simulink model "assignment4"  (R2014a)
settings: Solver=VariableStepDiscrete  StartTime=0.0  StopTime=100000  RelTol=1e-3
libraries: hdlsllib x20, simulink x10
settings Model: Creator=hirn.j  LastModifiedBy=you.r
settings OptimizationCC: BlockReduction=off  ConditionallyExecuteInputs=off  InlineParams=on
settings DebuggingCC: AlgebraicLoopMsg=error
settings HardwareCC: ProdHWDeviceType=ASIC/FPGA->ASIC/FPGA  ProdEqTarget=off

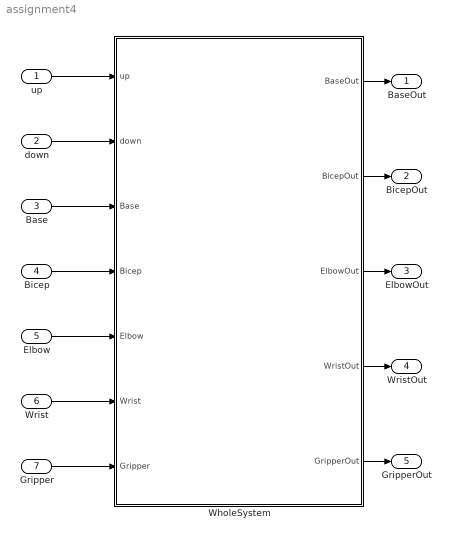
== system assignment4 ==
  up : Inport  OutDataTypeStr=boolean  SampleTime=1
  down : Inport  Port=2  OutDataTypeStr=boolean  SampleTime=1
  Base : Inport  Port=3  OutDataTypeStr=boolean  SampleTime=1
  Bicep : Inport  Port=4  OutDataTypeStr=boolean  SampleTime=1
  Elbow : Inport  Port=5  OutDataTypeStr=boolean  SampleTime=1
  Wrist : Inport  Port=6  OutDataTypeStr=boolean  SampleTime=1
  Gripper : Inport  Port=7  OutDataTypeStr=boolean  SampleTime=1
  WholeSystem : Subsystem  TreatAsAtomicUnit=on  SystemSampleTime=1
  BaseOut : Outport  SampleTime=1
  BicepOut : Outport  Port=2  SampleTime=1
  ElbowOut : Outport  Port=3  SampleTime=1
  WristOut : Outport  Port=4  SampleTime=1
  GripperOut : Outport  Port=5  SampleTime=1
  wires:
  up/1 -> WholeSystem/1(up)
  down/1 -> WholeSystem/2(down)
  Base/1 -> WholeSystem/3(Base)
  Bicep/1 -> WholeSystem/4(Bicep)
  Elbow/1 -> WholeSystem/5(Elbow)
  Wrist/1 -> WholeSystem/6(Wrist)
  Gripper/1 -> WholeSystem/7(Gripper)
  WholeSystem/1(BaseOut) -> BaseOut/1
  WholeSystem/2(BicepOut) -> BicepOut/1
  WholeSystem/3(ElbowOut) -> ElbowOut/1
  WholeSystem/4(WristOut) -> WristOut/1
  WholeSystem/5(GripperOut) -> GripperOut/1

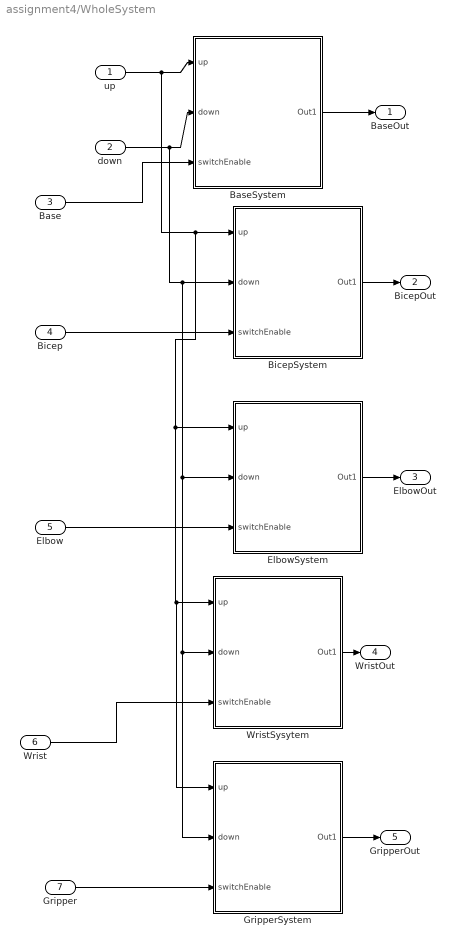
== system assignment4/WholeSystem ==
  up : Inport  OutDataTypeStr=boolean  SampleTime=1
  down : Inport  Port=2  OutDataTypeStr=boolean  SampleTime=1
  Base : Inport  Port=3  OutDataTypeStr=boolean  SampleTime=1
  Bicep : Inport  Port=4  OutDataTypeStr=boolean  SampleTime=1
  Elbow : Inport  Port=5  OutDataTypeStr=boolean  SampleTime=1
  Wrist : Inport  Port=6  OutDataTypeStr=boolean  SampleTime=1
  Gripper : Inport  Port=7  OutDataTypeStr=boolean  SampleTime=1
  BaseSystem : Subsystem  TreatAsAtomicUnit=on  SystemSampleTime=1
  BicepSystem : Subsystem  TreatAsAtomicUnit=on  SystemSampleTime=1
  ElbowSystem : Subsystem  TreatAsAtomicUnit=on  SystemSampleTime=1
  GripperSystem : Subsystem  TreatAsAtomicUnit=on  SystemSampleTime=1
  WristSysytem : Subsystem  TreatAsAtomicUnit=on  SystemSampleTime=1
  BaseOut : Outport  SampleTime=1
  BicepOut : Outport  Port=2  SampleTime=1
  ElbowOut : Outport  Port=3  SampleTime=1
  WristOut : Outport  Port=4  SampleTime=1
  GripperOut : Outport  Port=5  SampleTime=1
  wires:
  GripperSystem/1(Out1) -> GripperOut/1
  Bicep/1 -> BicepSystem/3(switchEnable)
  Base/1 -> BaseSystem/3(switchEnable)
  Wrist/1 -> WristSysytem/3(switchEnable)
  Elbow/1 -> ElbowSystem/3(switchEnable)
  Gripper/1 -> GripperSystem/3(switchEnable)
  up/1 -> GripperSystem/1(up), WristSysytem/1(up), ElbowSystem/1(up), BicepSystem/1(up), BaseSystem/1(up)
  down/1 -> GripperSystem/2(down), WristSysytem/2(down), ElbowSystem/2(down), BicepSystem/2(down), BaseSystem/2(down)
  BaseSystem/1(Out1) -> BaseOut/1
  BicepSystem/1(Out1) -> BicepOut/1
  WristSysytem/1(Out1) -> WristOut/1
  ElbowSystem/1(Out1) -> ElbowOut/1

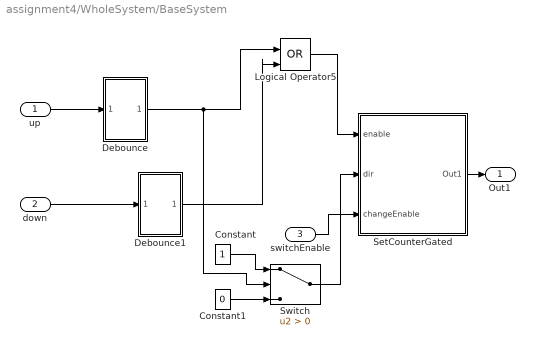
== system assignment4/WholeSystem/BaseSystem ==
  up : Inport  OutDataTypeStr=boolean  SampleTime=1
  down : Inport  Port=2  OutDataTypeStr=boolean  SampleTime=1
  switchEnable : Inport  Port=3  OutDataTypeStr=boolean  SampleTime=1
  Constant : Constant  OutDataTypeStr=boolean
  Constant1 : Constant  Value=0  OutDataTypeStr=boolean
  Debounce : Subsystem
  Debounce1 : Subsystem
  Logical Operator5 : Logic  Operator=OR  IconShape=distinctive  AllPortsSameDT=off  OutDataTypeStr=boolean  SampleTime=1
  SetCounterGated : Subsystem
  Switch : Switch  Criteria=u2 > Threshold
  Out1 : Outport  SampleTime=1
  wires:
  Debounce/1(Out1) -> Switch/2, Logical Operator5/1
  Logical Operator5/1 -> SetCounterGated/1(enable)
  up/1 -> Debounce/1(In1)
  down/1 -> Debounce1/1(In1)
  Constant/1 -> Switch/1
  Switch/1 -> SetCounterGated/2(dir)
  Constant1/1 -> Switch/3
  Debounce1/1(Out1) -> Logical Operator5/2
  SetCounterGated/1(Out1) -> Out1/1
  switchEnable/1 -> SetCounterGated/3(changeEnable)

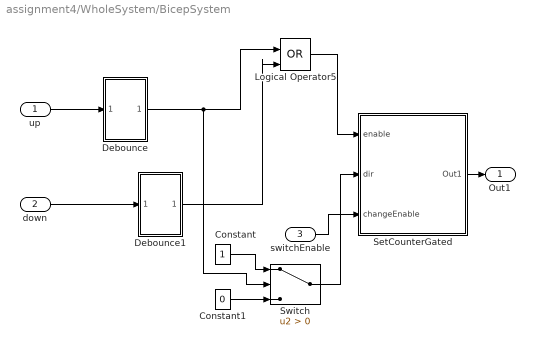
== system assignment4/WholeSystem/BicepSystem ==
  up : Inport  OutDataTypeStr=boolean  SampleTime=1
  down : Inport  Port=2  OutDataTypeStr=boolean  SampleTime=1
  switchEnable : Inport  Port=3  OutDataTypeStr=boolean  SampleTime=1
  Constant : Constant  OutDataTypeStr=boolean
  Constant1 : Constant  Value=0  OutDataTypeStr=boolean
  Debounce : Subsystem
  Debounce1 : Subsystem
  Logical Operator5 : Logic  Operator=OR  IconShape=distinctive  AllPortsSameDT=off  OutDataTypeStr=boolean  SampleTime=1
  SetCounterGated : Subsystem
  Switch : Switch  Criteria=u2 > Threshold
  Out1 : Outport  SampleTime=1
  wires:
  Debounce/1(Out1) -> Switch/2, Logical Operator5/1
  Logical Operator5/1 -> SetCounterGated/1(enable)
  up/1 -> Debounce/1(In1)
  down/1 -> Debounce1/1(In1)
  Constant/1 -> Switch/1
  Switch/1 -> SetCounterGated/2(dir)
  Constant1/1 -> Switch/3
  Debounce1/1(Out1) -> Logical Operator5/2
  SetCounterGated/1(Out1) -> Out1/1
  switchEnable/1 -> SetCounterGated/3(changeEnable)

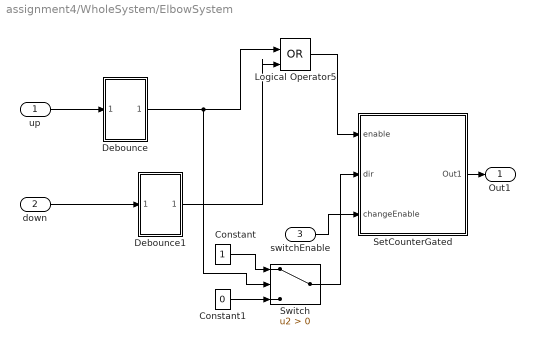
== system assignment4/WholeSystem/ElbowSystem ==
  up : Inport  OutDataTypeStr=boolean  SampleTime=1
  down : Inport  Port=2  OutDataTypeStr=boolean  SampleTime=1
  switchEnable : Inport  Port=3  OutDataTypeStr=boolean  SampleTime=1
  Constant : Constant  OutDataTypeStr=boolean
  Constant1 : Constant  Value=0  OutDataTypeStr=boolean
  Debounce : Subsystem
  Debounce1 : Subsystem
  Logical Operator5 : Logic  Operator=OR  IconShape=distinctive  AllPortsSameDT=off  OutDataTypeStr=boolean  SampleTime=1
  SetCounterGated : Subsystem
  Switch : Switch  Criteria=u2 > Threshold
  Out1 : Outport  SampleTime=1
  wires:
  Debounce/1(Out1) -> Switch/2, Logical Operator5/1
  Logical Operator5/1 -> SetCounterGated/1(enable)
  up/1 -> Debounce/1(In1)
  down/1 -> Debounce1/1(In1)
  Constant/1 -> Switch/1
  Switch/1 -> SetCounterGated/2(dir)
  Constant1/1 -> Switch/3
  Debounce1/1(Out1) -> Logical Operator5/2
  SetCounterGated/1(Out1) -> Out1/1
  switchEnable/1 -> SetCounterGated/3(changeEnable)

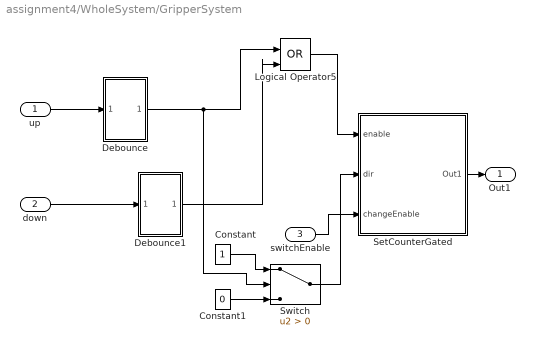
== system assignment4/WholeSystem/GripperSystem ==
  up : Inport  OutDataTypeStr=boolean  SampleTime=1
  down : Inport  Port=2  OutDataTypeStr=boolean  SampleTime=1
  switchEnable : Inport  Port=3  OutDataTypeStr=boolean  SampleTime=1
  Constant : Constant  OutDataTypeStr=boolean
  Constant1 : Constant  Value=0  OutDataTypeStr=boolean
  Debounce : Subsystem
  Debounce1 : Subsystem
  Logical Operator5 : Logic  Operator=OR  IconShape=distinctive  AllPortsSameDT=off  OutDataTypeStr=boolean  SampleTime=1
  SetCounterGated : Subsystem
  Switch : Switch  Criteria=u2 > Threshold
  Out1 : Outport  SampleTime=1
  wires:
  Debounce/1(Out1) -> Switch/2, Logical Operator5/1
  Logical Operator5/1 -> SetCounterGated/1(enable)
  up/1 -> Debounce/1(In1)
  down/1 -> Debounce1/1(In1)
  Constant/1 -> Switch/1
  Switch/1 -> SetCounterGated/2(dir)
  Constant1/1 -> Switch/3
  Debounce1/1(Out1) -> Logical Operator5/2
  SetCounterGated/1(Out1) -> Out1/1
  switchEnable/1 -> SetCounterGated/3(changeEnable)

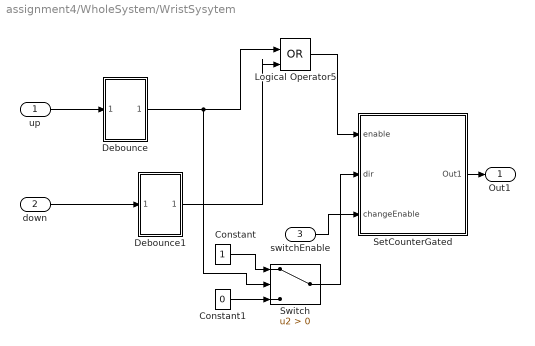
== system assignment4/WholeSystem/WristSysytem ==
  up : Inport  OutDataTypeStr=boolean  SampleTime=1
  down : Inport  Port=2  OutDataTypeStr=boolean  SampleTime=1
  switchEnable : Inport  Port=3  OutDataTypeStr=boolean  SampleTime=1
  Constant : Constant  OutDataTypeStr=boolean
  Constant1 : Constant  Value=0  OutDataTypeStr=boolean
  Debounce : Subsystem
  Debounce1 : Subsystem
  Logical Operator5 : Logic  Operator=OR  IconShape=distinctive  AllPortsSameDT=off  OutDataTypeStr=boolean  SampleTime=1
  SetCounterGated : Subsystem
  Switch : Switch  Criteria=u2 > Threshold
  Out1 : Outport  SampleTime=1
  wires:
  Debounce/1(Out1) -> Switch/2, Logical Operator5/1
  Logical Operator5/1 -> SetCounterGated/1(enable)
  up/1 -> Debounce/1(In1)
  down/1 -> Debounce1/1(In1)
  Constant/1 -> Switch/1
  Switch/1 -> SetCounterGated/2(dir)
  Constant1/1 -> Switch/3
  Debounce1/1(Out1) -> Logical Operator5/2
  SetCounterGated/1(Out1) -> Out1/1
  switchEnable/1 -> SetCounterGated/3(changeEnable)

== system assignment4/WholeSystem/BaseSystem/Debounce ==
  In1 : Inport
  Compare To Constant2 : simulink/Logic and Bit Operations/Compare To Constant  relop===  const=12500000  OutDataTypeStr=boolean
  Data Type Conversion1 : DataTypeConversion  OutDataTypeStr=boolean
  HDL Counter4 : hdlsllib/HDL Operations/HDL Counter  CountType=Free running  CountInit=0  CountStep=1  CountMax=100  CountFromType=Initial value  CountFrom=0  CountResetPort=on  CountLoadPort=off  CountEnbPort=on  CountDirPort=off  CountDataType=Unsigned  CountWordLen=32  CountFracLen=0  CountSampTime=1
  Logical Operator1 : Logic  Operator=NOT  IconShape=distinctive  AllPortsSameDT=off  OutDataTypeStr=boolean  SampleTime=1
  Out1 : Outport
  wires:
  Logical Operator1/1 -> HDL Counter4/1
  Compare To Constant2/1 -> Data Type Conversion1/1
  In1/1 -> HDL Counter4/2, Logical Operator1/1
  Data Type Conversion1/1 -> Out1/1
  HDL Counter4/1 -> Compare To Constant2/1

== system assignment4/WholeSystem/BaseSystem/Debounce1 ==
  In1 : Inport
  Compare To Constant2 : simulink/Logic and Bit Operations/Compare To Constant  relop===  const=12500000  OutDataTypeStr=boolean
  Data Type Conversion1 : DataTypeConversion  OutDataTypeStr=boolean
  HDL Counter4 : hdlsllib/HDL Operations/HDL Counter  CountType=Free running  CountInit=0  CountStep=1  CountMax=100  CountFromType=Initial value  CountFrom=0  CountResetPort=on  CountLoadPort=off  CountEnbPort=on  CountDirPort=off  CountDataType=Unsigned  CountWordLen=32  CountFracLen=0  CountSampTime=1
  Logical Operator1 : Logic  Operator=NOT  IconShape=distinctive  AllPortsSameDT=off  OutDataTypeStr=boolean  SampleTime=1
  Out1 : Outport
  wires:
  Logical Operator1/1 -> HDL Counter4/1
  Compare To Constant2/1 -> Data Type Conversion1/1
  In1/1 -> HDL Counter4/2, Logical Operator1/1
  Data Type Conversion1/1 -> Out1/1
  HDL Counter4/1 -> Compare To Constant2/1

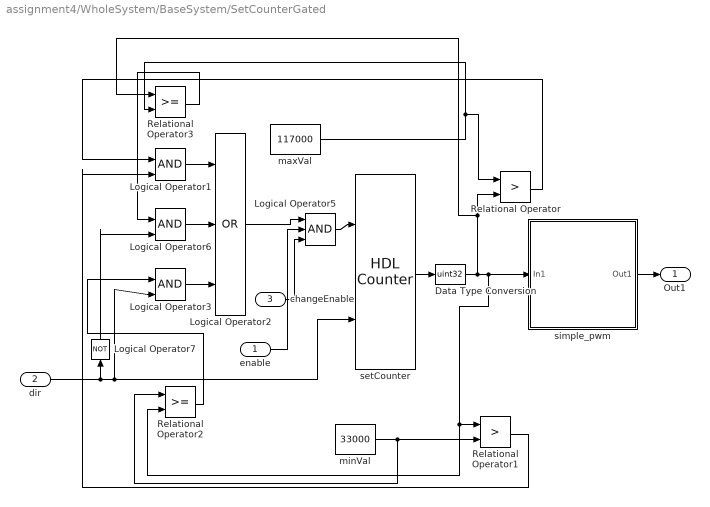
== system assignment4/WholeSystem/BaseSystem/SetCounterGated ==
  enable : Inport  OutDataTypeStr=boolean
  dir : Inport  Port=2  OutDataTypeStr=boolean
  changeEnable : Inport  Port=3  OutDataTypeStr=boolean
  Data Type Conversion : DataTypeConversion  OutDataTypeStr=uint32
  Logical Operator1 : Logic  IconShape=distinctive  AllPortsSameDT=off  OutDataTypeStr=boolean  SampleTime=1
  Logical Operator2 : Logic  Operator=OR  Inputs=3  IconShape=distinctive  AllPortsSameDT=off  OutDataTypeStr=boolean  SampleTime=1
  Logical Operator3 : Logic  IconShape=distinctive  AllPortsSameDT=off  OutDataTypeStr=boolean  SampleTime=1
  Logical Operator5 : Logic  Inputs=3  IconShape=distinctive  AllPortsSameDT=off  OutDataTypeStr=boolean  SampleTime=1
  Logical Operator6 : Logic  IconShape=distinctive  AllPortsSameDT=off  OutDataTypeStr=boolean  SampleTime=1
  Logical Operator7 : Logic  Operator=NOT  IconShape=distinctive  AllPortsSameDT=off  OutDataTypeStr=boolean  SampleTime=1
  Relational Operator : RelationalOperator  Operator=>  OutDataTypeStr=boolean
  Relational Operator1 : RelationalOperator  Operator=>  OutDataTypeStr=boolean
  Relational Operator2 : RelationalOperator  OutDataTypeStr=boolean
  Relational Operator3 : RelationalOperator  OutDataTypeStr=boolean
  maxVal : Constant  Value=117000  OutDataTypeStr=uint32
  minVal : Constant  Value=33000  OutDataTypeStr=uint32
  setCounter : hdlsllib/HDL Operations/HDL Counter  CountType=Count limited  CountInit=75000  CountStep=6000  CountMax=120000  CountFromType=Specify  CountFrom=30000  CountResetPort=off  CountLoadPort=off  CountEnbPort=on  CountDirPort=on  CountDataType=Unsigned  CountWordLen=20  CountFracLen=0  CountSampTime=1
  simple_pwm : Subsystem
  Out1 : Outport
  wires:
  Logical Operator7/1 -> Logical Operator6/2
  enable/1 -> Logical Operator5/2
  dir/1 -> Logical Operator7/1, Logical Operator3/2, setCounter/2
  setCounter/1 -> Data Type Conversion/1
  Logical Operator1/1 -> Logical Operator2/1
  Relational Operator/1 -> Logical Operator1/1
  maxVal/1 -> Relational Operator3/2, Relational Operator/1
  Logical Operator5/1 -> setCounter/1
  Relational Operator1/1 -> Logical Operator1/2
  Logical Operator2/1 -> Logical Operator5/1
  Logical Operator6/1 -> Logical Operator2/2
  Logical Operator3/1 -> Logical Operator2/3
  simple_pwm/1(Out1) -> Out1/1
  Data Type Conversion/1 -> Relational Operator2/2, Relational Operator1/1, simple_pwm/1(In1), Relational Operator3/1, Relational Operator/2
  minVal/1 -> Relational Operator2/1, Relational Operator1/2
  Relational Operator2/1 -> Logical Operator3/1
  Relational Operator3/1 -> Logical Operator6/1
  changeEnable/1 -> Logical Operator5/3

== system assignment4/WholeSystem/BicepSystem/Debounce ==
  In1 : Inport
  Compare To Constant2 : simulink/Logic and Bit Operations/Compare To Constant  relop===  const=12500000  OutDataTypeStr=boolean
  Data Type Conversion1 : DataTypeConversion  OutDataTypeStr=boolean
  HDL Counter4 : hdlsllib/HDL Operations/HDL Counter  CountType=Free running  CountInit=0  CountStep=1  CountMax=100  CountFromType=Initial value  CountFrom=0  CountResetPort=on  CountLoadPort=off  CountEnbPort=on  CountDirPort=off  CountDataType=Unsigned  CountWordLen=32  CountFracLen=0  CountSampTime=1
  Logical Operator1 : Logic  Operator=NOT  IconShape=distinctive  AllPortsSameDT=off  OutDataTypeStr=boolean  SampleTime=1
  Out1 : Outport
  wires:
  Logical Operator1/1 -> HDL Counter4/1
  Compare To Constant2/1 -> Data Type Conversion1/1
  In1/1 -> HDL Counter4/2, Logical Operator1/1
  Data Type Conversion1/1 -> Out1/1
  HDL Counter4/1 -> Compare To Constant2/1

== system assignment4/WholeSystem/BicepSystem/Debounce1 ==
  In1 : Inport
  Compare To Constant2 : simulink/Logic and Bit Operations/Compare To Constant  relop===  const=12500000  OutDataTypeStr=boolean
  Data Type Conversion1 : DataTypeConversion  OutDataTypeStr=boolean
  HDL Counter4 : hdlsllib/HDL Operations/HDL Counter  CountType=Free running  CountInit=0  CountStep=1  CountMax=100  CountFromType=Initial value  CountFrom=0  CountResetPort=on  CountLoadPort=off  CountEnbPort=on  CountDirPort=off  CountDataType=Unsigned  CountWordLen=32  CountFracLen=0  CountSampTime=1
  Logical Operator1 : Logic  Operator=NOT  IconShape=distinctive  AllPortsSameDT=off  OutDataTypeStr=boolean  SampleTime=1
  Out1 : Outport
  wires:
  Logical Operator1/1 -> HDL Counter4/1
  Compare To Constant2/1 -> Data Type Conversion1/1
  In1/1 -> HDL Counter4/2, Logical Operator1/1
  Data Type Conversion1/1 -> Out1/1
  HDL Counter4/1 -> Compare To Constant2/1

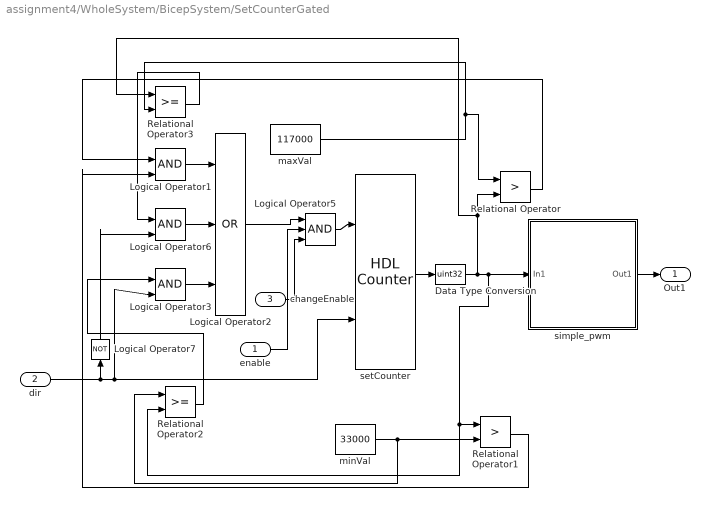
== system assignment4/WholeSystem/BicepSystem/SetCounterGated ==
  enable : Inport  OutDataTypeStr=boolean
  dir : Inport  Port=2  OutDataTypeStr=boolean
  changeEnable : Inport  Port=3  OutDataTypeStr=boolean
  Data Type Conversion : DataTypeConversion  OutDataTypeStr=uint32
  Logical Operator1 : Logic  IconShape=distinctive  AllPortsSameDT=off  OutDataTypeStr=boolean  SampleTime=1
  Logical Operator2 : Logic  Operator=OR  Inputs=3  IconShape=distinctive  AllPortsSameDT=off  OutDataTypeStr=boolean  SampleTime=1
  Logical Operator3 : Logic  IconShape=distinctive  AllPortsSameDT=off  OutDataTypeStr=boolean  SampleTime=1
  Logical Operator5 : Logic  Inputs=3  IconShape=distinctive  AllPortsSameDT=off  OutDataTypeStr=boolean  SampleTime=1
  Logical Operator6 : Logic  IconShape=distinctive  AllPortsSameDT=off  OutDataTypeStr=boolean  SampleTime=1
  Logical Operator7 : Logic  Operator=NOT  IconShape=distinctive  AllPortsSameDT=off  OutDataTypeStr=boolean  SampleTime=1
  Relational Operator : RelationalOperator  Operator=>  OutDataTypeStr=boolean
  Relational Operator1 : RelationalOperator  Operator=>  OutDataTypeStr=boolean
  Relational Operator2 : RelationalOperator  OutDataTypeStr=boolean
  Relational Operator3 : RelationalOperator  OutDataTypeStr=boolean
  maxVal : Constant  Value=117000  OutDataTypeStr=uint32
  minVal : Constant  Value=33000  OutDataTypeStr=uint32
  setCounter : hdlsllib/HDL Operations/HDL Counter  CountType=Count limited  CountInit=75000  CountStep=6000  CountMax=120000  CountFromType=Specify  CountFrom=30000  CountResetPort=off  CountLoadPort=off  CountEnbPort=on  CountDirPort=on  CountDataType=Unsigned  CountWordLen=20  CountFracLen=0  CountSampTime=1
  simple_pwm : Subsystem
  Out1 : Outport
  wires:
  Logical Operator7/1 -> Logical Operator6/2
  enable/1 -> Logical Operator5/2
  dir/1 -> Logical Operator7/1, Logical Operator3/2, setCounter/2
  setCounter/1 -> Data Type Conversion/1
  Logical Operator1/1 -> Logical Operator2/1
  Relational Operator/1 -> Logical Operator1/1
  maxVal/1 -> Relational Operator3/2, Relational Operator/1
  Logical Operator5/1 -> setCounter/1
  Relational Operator1/1 -> Logical Operator1/2
  Logical Operator2/1 -> Logical Operator5/1
  Logical Operator6/1 -> Logical Operator2/2
  Logical Operator3/1 -> Logical Operator2/3
  simple_pwm/1(Out1) -> Out1/1
  Data Type Conversion/1 -> Relational Operator2/2, Relational Operator1/1, simple_pwm/1(In1), Relational Operator3/1, Relational Operator/2
  minVal/1 -> Relational Operator2/1, Relational Operator1/2
  Relational Operator2/1 -> Logical Operator3/1
  Relational Operator3/1 -> Logical Operator6/1
  changeEnable/1 -> Logical Operator5/3

== system assignment4/WholeSystem/ElbowSystem/Debounce ==
  In1 : Inport
  Compare To Constant2 : simulink/Logic and Bit Operations/Compare To Constant  relop===  const=12500000  OutDataTypeStr=boolean
  Data Type Conversion1 : DataTypeConversion  OutDataTypeStr=boolean
  HDL Counter4 : hdlsllib/HDL Operations/HDL Counter  CountType=Free running  CountInit=0  CountStep=1  CountMax=100  CountFromType=Initial value  CountFrom=0  CountResetPort=on  CountLoadPort=off  CountEnbPort=on  CountDirPort=off  CountDataType=Unsigned  CountWordLen=32  CountFracLen=0  CountSampTime=1
  Logical Operator1 : Logic  Operator=NOT  IconShape=distinctive  AllPortsSameDT=off  OutDataTypeStr=boolean  SampleTime=1
  Out1 : Outport
  wires:
  Logical Operator1/1 -> HDL Counter4/1
  Compare To Constant2/1 -> Data Type Conversion1/1
  In1/1 -> HDL Counter4/2, Logical Operator1/1
  Data Type Conversion1/1 -> Out1/1
  HDL Counter4/1 -> Compare To Constant2/1

== system assignment4/WholeSystem/ElbowSystem/Debounce1 ==
  In1 : Inport
  Compare To Constant2 : simulink/Logic and Bit Operations/Compare To Constant  relop===  const=12500000  OutDataTypeStr=boolean
  Data Type Conversion1 : DataTypeConversion  OutDataTypeStr=boolean
  HDL Counter4 : hdlsllib/HDL Operations/HDL Counter  CountType=Free running  CountInit=0  CountStep=1  CountMax=100  CountFromType=Initial value  CountFrom=0  CountResetPort=on  CountLoadPort=off  CountEnbPort=on  CountDirPort=off  CountDataType=Unsigned  CountWordLen=32  CountFracLen=0  CountSampTime=1
  Logical Operator1 : Logic  Operator=NOT  IconShape=distinctive  AllPortsSameDT=off  OutDataTypeStr=boolean  SampleTime=1
  Out1 : Outport
  wires:
  Logical Operator1/1 -> HDL Counter4/1
  Compare To Constant2/1 -> Data Type Conversion1/1
  In1/1 -> HDL Counter4/2, Logical Operator1/1
  Data Type Conversion1/1 -> Out1/1
  HDL Counter4/1 -> Compare To Constant2/1

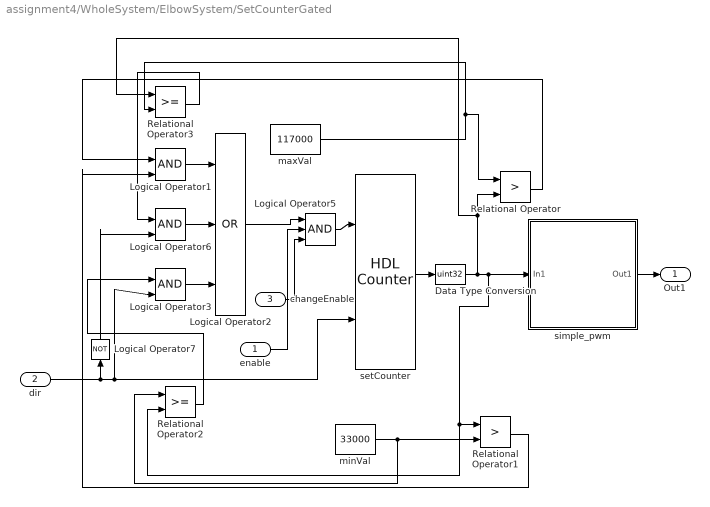
== system assignment4/WholeSystem/ElbowSystem/SetCounterGated ==
  enable : Inport  OutDataTypeStr=boolean
  dir : Inport  Port=2  OutDataTypeStr=boolean
  changeEnable : Inport  Port=3  OutDataTypeStr=boolean
  Data Type Conversion : DataTypeConversion  OutDataTypeStr=uint32
  Logical Operator1 : Logic  IconShape=distinctive  AllPortsSameDT=off  OutDataTypeStr=boolean  SampleTime=1
  Logical Operator2 : Logic  Operator=OR  Inputs=3  IconShape=distinctive  AllPortsSameDT=off  OutDataTypeStr=boolean  SampleTime=1
  Logical Operator3 : Logic  IconShape=distinctive  AllPortsSameDT=off  OutDataTypeStr=boolean  SampleTime=1
  Logical Operator5 : Logic  Inputs=3  IconShape=distinctive  AllPortsSameDT=off  OutDataTypeStr=boolean  SampleTime=1
  Logical Operator6 : Logic  IconShape=distinctive  AllPortsSameDT=off  OutDataTypeStr=boolean  SampleTime=1
  Logical Operator7 : Logic  Operator=NOT  IconShape=distinctive  AllPortsSameDT=off  OutDataTypeStr=boolean  SampleTime=1
  Relational Operator : RelationalOperator  Operator=>  OutDataTypeStr=boolean
  Relational Operator1 : RelationalOperator  Operator=>  OutDataTypeStr=boolean
  Relational Operator2 : RelationalOperator  OutDataTypeStr=boolean
  Relational Operator3 : RelationalOperator  OutDataTypeStr=boolean
  maxVal : Constant  Value=117000  OutDataTypeStr=uint32
  minVal : Constant  Value=33000  OutDataTypeStr=uint32
  setCounter : hdlsllib/HDL Operations/HDL Counter  CountType=Count limited  CountInit=75000  CountStep=6000  CountMax=120000  CountFromType=Specify  CountFrom=30000  CountResetPort=off  CountLoadPort=off  CountEnbPort=on  CountDirPort=on  CountDataType=Unsigned  CountWordLen=20  CountFracLen=0  CountSampTime=1
  simple_pwm : Subsystem
  Out1 : Outport
  wires:
  Logical Operator7/1 -> Logical Operator6/2
  enable/1 -> Logical Operator5/2
  dir/1 -> Logical Operator7/1, Logical Operator3/2, setCounter/2
  setCounter/1 -> Data Type Conversion/1
  Logical Operator1/1 -> Logical Operator2/1
  Relational Operator/1 -> Logical Operator1/1
  maxVal/1 -> Relational Operator3/2, Relational Operator/1
  Logical Operator5/1 -> setCounter/1
  Relational Operator1/1 -> Logical Operator1/2
  Logical Operator2/1 -> Logical Operator5/1
  Logical Operator6/1 -> Logical Operator2/2
  Logical Operator3/1 -> Logical Operator2/3
  simple_pwm/1(Out1) -> Out1/1
  Data Type Conversion/1 -> Relational Operator2/2, Relational Operator1/1, simple_pwm/1(In1), Relational Operator3/1, Relational Operator/2
  minVal/1 -> Relational Operator2/1, Relational Operator1/2
  Relational Operator2/1 -> Logical Operator3/1
  Relational Operator3/1 -> Logical Operator6/1
  changeEnable/1 -> Logical Operator5/3

== system assignment4/WholeSystem/GripperSystem/Debounce ==
  In1 : Inport
  Compare To Constant2 : simulink/Logic and Bit Operations/Compare To Constant  relop===  const=12500000  OutDataTypeStr=boolean
  Data Type Conversion1 : DataTypeConversion  OutDataTypeStr=boolean
  HDL Counter4 : hdlsllib/HDL Operations/HDL Counter  CountType=Free running  CountInit=0  CountStep=1  CountMax=100  CountFromType=Initial value  CountFrom=0  CountResetPort=on  CountLoadPort=off  CountEnbPort=on  CountDirPort=off  CountDataType=Unsigned  CountWordLen=32  CountFracLen=0  CountSampTime=1
  Logical Operator1 : Logic  Operator=NOT  IconShape=distinctive  AllPortsSameDT=off  OutDataTypeStr=boolean  SampleTime=1
  Out1 : Outport
  wires:
  Logical Operator1/1 -> HDL Counter4/1
  Compare To Constant2/1 -> Data Type Conversion1/1
  In1/1 -> HDL Counter4/2, Logical Operator1/1
  Data Type Conversion1/1 -> Out1/1
  HDL Counter4/1 -> Compare To Constant2/1

== system assignment4/WholeSystem/GripperSystem/Debounce1 ==
  In1 : Inport
  Compare To Constant2 : simulink/Logic and Bit Operations/Compare To Constant  relop===  const=12500000  OutDataTypeStr=boolean
  Data Type Conversion1 : DataTypeConversion  OutDataTypeStr=boolean
  HDL Counter4 : hdlsllib/HDL Operations/HDL Counter  CountType=Free running  CountInit=0  CountStep=1  CountMax=100  CountFromType=Initial value  CountFrom=0  CountResetPort=on  CountLoadPort=off  CountEnbPort=on  CountDirPort=off  CountDataType=Unsigned  CountWordLen=32  CountFracLen=0  CountSampTime=1
  Logical Operator1 : Logic  Operator=NOT  IconShape=distinctive  AllPortsSameDT=off  OutDataTypeStr=boolean  SampleTime=1
  Out1 : Outport
  wires:
  Logical Operator1/1 -> HDL Counter4/1
  Compare To Constant2/1 -> Data Type Conversion1/1
  In1/1 -> HDL Counter4/2, Logical Operator1/1
  Data Type Conversion1/1 -> Out1/1
  HDL Counter4/1 -> Compare To Constant2/1

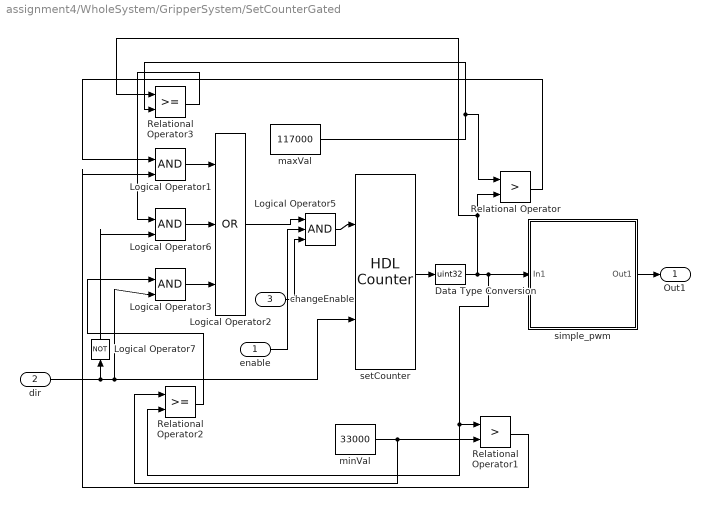
== system assignment4/WholeSystem/GripperSystem/SetCounterGated ==
  enable : Inport  OutDataTypeStr=boolean
  dir : Inport  Port=2  OutDataTypeStr=boolean
  changeEnable : Inport  Port=3  OutDataTypeStr=boolean
  Data Type Conversion : DataTypeConversion  OutDataTypeStr=uint32
  Logical Operator1 : Logic  IconShape=distinctive  AllPortsSameDT=off  OutDataTypeStr=boolean  SampleTime=1
  Logical Operator2 : Logic  Operator=OR  Inputs=3  IconShape=distinctive  AllPortsSameDT=off  OutDataTypeStr=boolean  SampleTime=1
  Logical Operator3 : Logic  IconShape=distinctive  AllPortsSameDT=off  OutDataTypeStr=boolean  SampleTime=1
  Logical Operator5 : Logic  Inputs=3  IconShape=distinctive  AllPortsSameDT=off  OutDataTypeStr=boolean  SampleTime=1
  Logical Operator6 : Logic  IconShape=distinctive  AllPortsSameDT=off  OutDataTypeStr=boolean  SampleTime=1
  Logical Operator7 : Logic  Operator=NOT  IconShape=distinctive  AllPortsSameDT=off  OutDataTypeStr=boolean  SampleTime=1
  Relational Operator : RelationalOperator  Operator=>  OutDataTypeStr=boolean
  Relational Operator1 : RelationalOperator  Operator=>  OutDataTypeStr=boolean
  Relational Operator2 : RelationalOperator  OutDataTypeStr=boolean
  Relational Operator3 : RelationalOperator  OutDataTypeStr=boolean
  maxVal : Constant  Value=117000  OutDataTypeStr=uint32
  minVal : Constant  Value=33000  OutDataTypeStr=uint32
  setCounter : hdlsllib/HDL Operations/HDL Counter  CountType=Count limited  CountInit=75000  CountStep=6000  CountMax=120000  CountFromType=Specify  CountFrom=30000  CountResetPort=off  CountLoadPort=off  CountEnbPort=on  CountDirPort=on  CountDataType=Unsigned  CountWordLen=20  CountFracLen=0  CountSampTime=1
  simple_pwm : Subsystem
  Out1 : Outport
  wires:
  Logical Operator7/1 -> Logical Operator6/2
  enable/1 -> Logical Operator5/2
  dir/1 -> Logical Operator7/1, Logical Operator3/2, setCounter/2
  setCounter/1 -> Data Type Conversion/1
  Logical Operator1/1 -> Logical Operator2/1
  Relational Operator/1 -> Logical Operator1/1
  maxVal/1 -> Relational Operator3/2, Relational Operator/1
  Logical Operator5/1 -> setCounter/1
  Relational Operator1/1 -> Logical Operator1/2
  Logical Operator2/1 -> Logical Operator5/1
  Logical Operator6/1 -> Logical Operator2/2
  Logical Operator3/1 -> Logical Operator2/3
  simple_pwm/1(Out1) -> Out1/1
  Data Type Conversion/1 -> Relational Operator2/2, Relational Operator1/1, simple_pwm/1(In1), Relational Operator3/1, Relational Operator/2
  minVal/1 -> Relational Operator2/1, Relational Operator1/2
  Relational Operator2/1 -> Logical Operator3/1
  Relational Operator3/1 -> Logical Operator6/1
  changeEnable/1 -> Logical Operator5/3

== system assignment4/WholeSystem/WristSysytem/Debounce ==
  In1 : Inport
  Compare To Constant2 : simulink/Logic and Bit Operations/Compare To Constant  relop===  const=12500000  OutDataTypeStr=boolean
  Data Type Conversion1 : DataTypeConversion  OutDataTypeStr=boolean
  HDL Counter4 : hdlsllib/HDL Operations/HDL Counter  CountType=Free running  CountInit=0  CountStep=1  CountMax=100  CountFromType=Initial value  CountFrom=0  CountResetPort=on  CountLoadPort=off  CountEnbPort=on  CountDirPort=off  CountDataType=Unsigned  CountWordLen=32  CountFracLen=0  CountSampTime=1
  Logical Operator1 : Logic  Operator=NOT  IconShape=distinctive  AllPortsSameDT=off  OutDataTypeStr=boolean  SampleTime=1
  Out1 : Outport
  wires:
  Logical Operator1/1 -> HDL Counter4/1
  Compare To Constant2/1 -> Data Type Conversion1/1
  In1/1 -> HDL Counter4/2, Logical Operator1/1
  Data Type Conversion1/1 -> Out1/1
  HDL Counter4/1 -> Compare To Constant2/1

== system assignment4/WholeSystem/WristSysytem/Debounce1 ==
  In1 : Inport
  Compare To Constant2 : simulink/Logic and Bit Operations/Compare To Constant  relop===  const=12500000  OutDataTypeStr=boolean
  Data Type Conversion1 : DataTypeConversion  OutDataTypeStr=boolean
  HDL Counter4 : hdlsllib/HDL Operations/HDL Counter  CountType=Free running  CountInit=0  CountStep=1  CountMax=100  CountFromType=Initial value  CountFrom=0  CountResetPort=on  CountLoadPort=off  CountEnbPort=on  CountDirPort=off  CountDataType=Unsigned  CountWordLen=32  CountFracLen=0  CountSampTime=1
  Logical Operator1 : Logic  Operator=NOT  IconShape=distinctive  AllPortsSameDT=off  OutDataTypeStr=boolean  SampleTime=1
  Out1 : Outport
  wires:
  Logical Operator1/1 -> HDL Counter4/1
  Compare To Constant2/1 -> Data Type Conversion1/1
  In1/1 -> HDL Counter4/2, Logical Operator1/1
  Data Type Conversion1/1 -> Out1/1
  HDL Counter4/1 -> Compare To Constant2/1

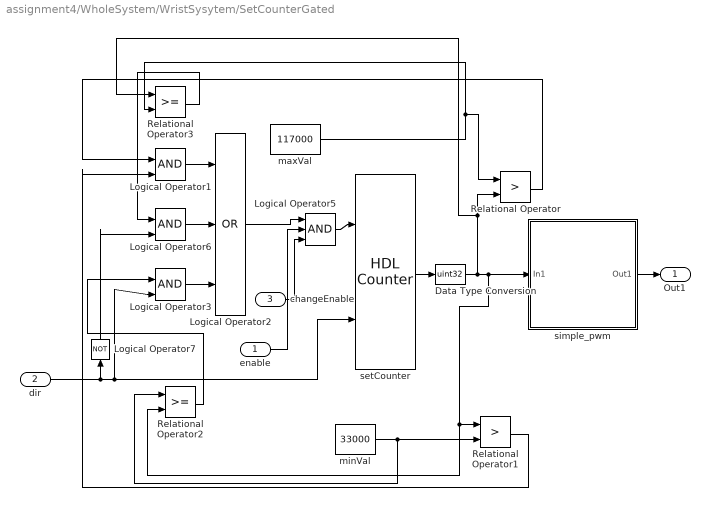
== system assignment4/WholeSystem/WristSysytem/SetCounterGated ==
  enable : Inport  OutDataTypeStr=boolean
  dir : Inport  Port=2  OutDataTypeStr=boolean
  changeEnable : Inport  Port=3  OutDataTypeStr=boolean
  Data Type Conversion : DataTypeConversion  OutDataTypeStr=uint32
  Logical Operator1 : Logic  IconShape=distinctive  AllPortsSameDT=off  OutDataTypeStr=boolean  SampleTime=1
  Logical Operator2 : Logic  Operator=OR  Inputs=3  IconShape=distinctive  AllPortsSameDT=off  OutDataTypeStr=boolean  SampleTime=1
  Logical Operator3 : Logic  IconShape=distinctive  AllPortsSameDT=off  OutDataTypeStr=boolean  SampleTime=1
  Logical Operator5 : Logic  Inputs=3  IconShape=distinctive  AllPortsSameDT=off  OutDataTypeStr=boolean  SampleTime=1
  Logical Operator6 : Logic  IconShape=distinctive  AllPortsSameDT=off  OutDataTypeStr=boolean  SampleTime=1
  Logical Operator7 : Logic  Operator=NOT  IconShape=distinctive  AllPortsSameDT=off  OutDataTypeStr=boolean  SampleTime=1
  Relational Operator : RelationalOperator  Operator=>  OutDataTypeStr=boolean
  Relational Operator1 : RelationalOperator  Operator=>  OutDataTypeStr=boolean
  Relational Operator2 : RelationalOperator  OutDataTypeStr=boolean
  Relational Operator3 : RelationalOperator  OutDataTypeStr=boolean
  maxVal : Constant  Value=117000  OutDataTypeStr=uint32
  minVal : Constant  Value=33000  OutDataTypeStr=uint32
  setCounter : hdlsllib/HDL Operations/HDL Counter  CountType=Count limited  CountInit=75000  CountStep=6000  CountMax=120000  CountFromType=Specify  CountFrom=30000  CountResetPort=off  CountLoadPort=off  CountEnbPort=on  CountDirPort=on  CountDataType=Unsigned  CountWordLen=20  CountFracLen=0  CountSampTime=1
  simple_pwm : Subsystem
  Out1 : Outport
  wires:
  Logical Operator7/1 -> Logical Operator6/2
  enable/1 -> Logical Operator5/2
  dir/1 -> Logical Operator7/1, Logical Operator3/2, setCounter/2
  setCounter/1 -> Data Type Conversion/1
  Logical Operator1/1 -> Logical Operator2/1
  Relational Operator/1 -> Logical Operator1/1
  maxVal/1 -> Relational Operator3/2, Relational Operator/1
  Logical Operator5/1 -> setCounter/1
  Relational Operator1/1 -> Logical Operator1/2
  Logical Operator2/1 -> Logical Operator5/1
  Logical Operator6/1 -> Logical Operator2/2
  Logical Operator3/1 -> Logical Operator2/3
  simple_pwm/1(Out1) -> Out1/1
  Data Type Conversion/1 -> Relational Operator2/2, Relational Operator1/1, simple_pwm/1(In1), Relational Operator3/1, Relational Operator/2
  minVal/1 -> Relational Operator2/1, Relational Operator1/2
  Relational Operator2/1 -> Logical Operator3/1
  Relational Operator3/1 -> Logical Operator6/1
  changeEnable/1 -> Logical Operator5/3

== system assignment4/WholeSystem/BaseSystem/SetCounterGated/simple_pwm ==
  In1 : Inport  OutDataTypeStr=uint32
  HDL Counter : hdlsllib/HDL Operations/HDL Counter  CountType=Count limited  CountInit=0  CountStep=1  CountMax=1000000  CountFromType=Initial value  CountFrom=0  CountResetPort=off  CountLoadPort=off  CountEnbPort=off  CountDirPort=off  CountDataType=Unsigned  CountWordLen=20  CountFracLen=0  CountSampTime=1
  Relational Operator : RelationalOperator  Operator=<  OutDataTypeStr=boolean  SampleTime=1
  Out1 : Outport
  wires:
  Relational Operator/1 -> Out1/1
  HDL Counter/1 -> Relational Operator/1
  In1/1 -> Relational Operator/2

== system assignment4/WholeSystem/BicepSystem/SetCounterGated/simple_pwm ==
  In1 : Inport  OutDataTypeStr=uint32
  HDL Counter : hdlsllib/HDL Operations/HDL Counter  CountType=Count limited  CountInit=0  CountStep=1  CountMax=1000000  CountFromType=Initial value  CountFrom=0  CountResetPort=off  CountLoadPort=off  CountEnbPort=off  CountDirPort=off  CountDataType=Unsigned  CountWordLen=20  CountFracLen=0  CountSampTime=1
  Relational Operator : RelationalOperator  Operator=<  OutDataTypeStr=boolean  SampleTime=1
  Out1 : Outport
  wires:
  Relational Operator/1 -> Out1/1
  HDL Counter/1 -> Relational Operator/1
  In1/1 -> Relational Operator/2

== system assignment4/WholeSystem/ElbowSystem/SetCounterGated/simple_pwm ==
  In1 : Inport  OutDataTypeStr=uint32
  HDL Counter : hdlsllib/HDL Operations/HDL Counter  CountType=Count limited  CountInit=0  CountStep=1  CountMax=1000000  CountFromType=Initial value  CountFrom=0  CountResetPort=off  CountLoadPort=off  CountEnbPort=off  CountDirPort=off  CountDataType=Unsigned  CountWordLen=20  CountFracLen=0  CountSampTime=1
  Relational Operator : RelationalOperator  Operator=<  OutDataTypeStr=boolean  SampleTime=1
  Out1 : Outport
  wires:
  Relational Operator/1 -> Out1/1
  HDL Counter/1 -> Relational Operator/1
  In1/1 -> Relational Operator/2

== system assignment4/WholeSystem/GripperSystem/SetCounterGated/simple_pwm ==
  In1 : Inport  OutDataTypeStr=uint32
  HDL Counter : hdlsllib/HDL Operations/HDL Counter  CountType=Count limited  CountInit=0  CountStep=1  CountMax=1000000  CountFromType=Initial value  CountFrom=0  CountResetPort=off  CountLoadPort=off  CountEnbPort=off  CountDirPort=off  CountDataType=Unsigned  CountWordLen=20  CountFracLen=0  CountSampTime=1
  Relational Operator : RelationalOperator  Operator=<  OutDataTypeStr=boolean  SampleTime=1
  Out1 : Outport
  wires:
  Relational Operator/1 -> Out1/1
  HDL Counter/1 -> Relational Operator/1
  In1/1 -> Relational Operator/2

== system assignment4/WholeSystem/WristSysytem/SetCounterGated/simple_pwm ==
  In1 : Inport  OutDataTypeStr=uint32
  HDL Counter : hdlsllib/HDL Operations/HDL Counter  CountType=Count limited  CountInit=0  CountStep=1  CountMax=1000000  CountFromType=Initial value  CountFrom=0  CountResetPort=off  CountLoadPort=off  CountEnbPort=off  CountDirPort=off  CountDataType=Unsigned  CountWordLen=20  CountFracLen=0  CountSampTime=1
  Relational Operator : RelationalOperator  Operator=<  OutDataTypeStr=boolean  SampleTime=1
  Out1 : Outport
  wires:
  Relational Operator/1 -> Out1/1
  HDL Counter/1 -> Relational Operator/1
  In1/1 -> Relational Operator/2
